simulink library "fiveDoFDynamicsCoupledFossenTurbDynamics"  (R2022a)
settings: Solver=VariableStepAuto  StartTime=0.0  StopTime=10.0  RelTol=1e-3
undefined symbols (not defined in the file): eulAng2RotMat_ul, eulDot, EulerAngle2RotMat, vcl
libraries: vrlib x7, sharedutil x3, posAng2RotMat_ul x1, elevAzimAngles x1
settings Model: Creator=jldanie5  LastModifiedBy=adabney
settings SolverCC: AlgebraicLoopSolver=TrustRegion
settings DebuggingCC: UnconnectedInputMsg=warning  UnconnectedOutputMsg=warning  UnconnectedLineMsg=warning  SFMachineParentedDataDiag=warning  ArithmeticOperatorsInVariantConditions=warning
settings SFSimCC: CustomCodeUndefinedFunction=UseInterfaceOnly

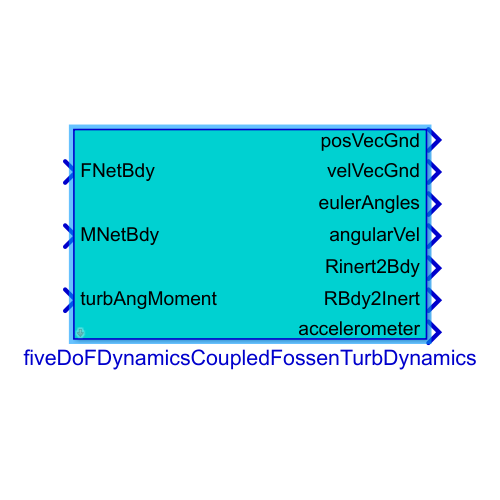
[thumbnail: Simulink's stored preview of the top-level diagram]
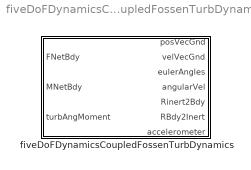
== system fiveDoFDynamicsCoupledFossenTurbDynamics ==
  fiveDoFDynamicsCoupledFossenTurbDynamics : Subsystem  VariantControl=VSS_sixDoFDynamics_sixDoFDynamicsCoupledFossenTurbDynamics  mask{MMat=vcl.M6x6_B.Value, MaMat=vcl.Ma6x6_LE.Value, rCM_B=vcl.rCM_B.Value, rB_LE=vcl.rB_LE.Value, initPos=vcl.initPosVecGnd.Value, initVel=vcl.initVelVecBdy.Value, initEulAngs=vcl.initEulAng.Value, initAngVel=vcl.initAngVelVec.Value}
      mask prompts: MMat "6x6 Mass Matrix"; MaMat "6x6 Added Mass Matrix"; rCM_B "Center of mass position vec in body frame"; rB_LE "Body frame origin position vec relative to Leading Edge"; initPos "Initial position"; initVel "Initial velocity"; initEulAngs "Initial Euler Angles"; initAngVel "Initial Angular Velocity Vec"
      mask init:
      | %Calculate Added Mass Matrices
      | S = @(v) [0 -v(3) v(2);v(3) 0 -v(1);-v(2) v(1) 0];
      | MaAdj = [eye(3) zeros(3);-S(rB_LE) eye(3)]*MaMat;
      | MTot = MMat + MaAdj;
      | MTotInv = inv(MTot);
      | 
      | %Calculate system mass and inertia
      | m = MMat(1,1);
      | J = MMat(4:6,4:6);%About Body Frame 
      | 
      | %Calculate system initial position angles
      | x = initPos(1);
      | y = initPos(2);
      | z = initPos(3);
      | R = sqrt(sum(initPos.^2));
      | el = atan2(z,sqrt(x^2+y^2));
      | az = atan2(y,x);
      | 
      | %Calculate initial spherical velocities
      | r = initEulAngs(1); sr = sin(r); cr = cos(r);
      | p = initEulAngs(2); sp = sin(p); cp = cos(p);
      | y = initEulAngs(3); sy = sin(y); cy = cos(y);
      | se = sin(el); ce = cos(el);
      | sa = sin(az); ca = cos(az);
      | 
      | %Calculate Rotation Matrices
      | Rx = [1 0 0; 0 cr sr; 0 -sr cr];
      | Ry = [cp 0 -sp; 0 1 0; sp 0 cp];
      | Rz = [cy sy 0; -sy cy 0; 0 0 1];
      | Ra = [ca sa 0; -sa ca 0; 0 0 1];
      | Re = [ce 0 -se; 0 1 0; se 0 ce];
      | Reul = Rx*Ry*Rz;
      | Rsph = Re*Ra;
      | 
      | %Calculate Initial Velocities
      | velSp = Rsph*Reul'*initVel;
      | initVelSph = velSp(2:3);
      mask DialogControl Container6 Prompt: Mass Matrices
      mask DialogControl Container4 Prompt: Point Locations
      mask DialogControl Container3 Prompt: Initial Conditions

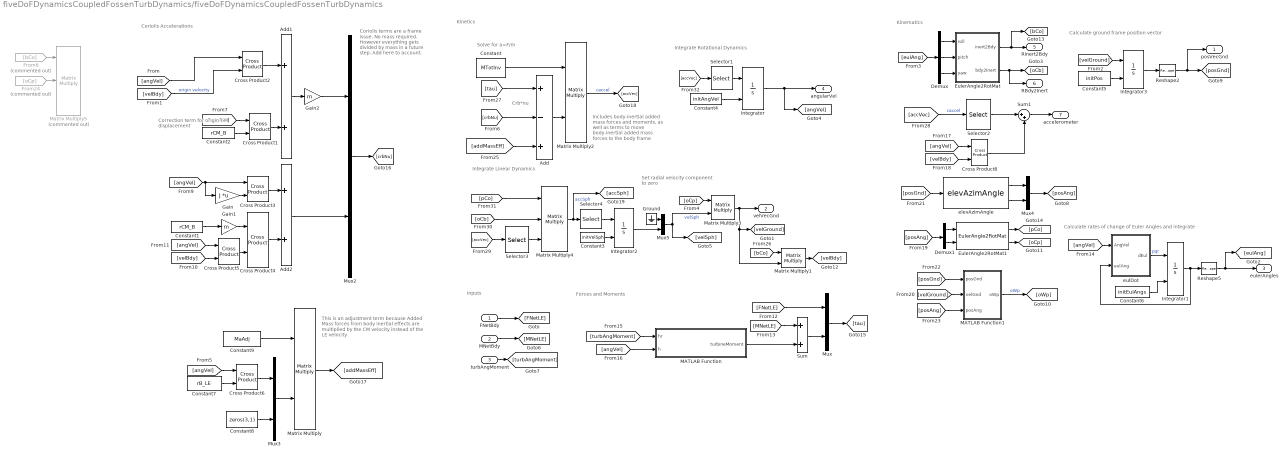
== system fiveDoFDynamicsCoupledFossenTurbDynamics/fiveDoFDynamicsCoupledFossenTurbDynamics ==
  note: Kinematics
  note: Kinetics
  note: Set radial velocity
      | component to zero
  note: Integrate Linear Dynamics
  note: Coriolis terms are a frame issue. No mass required. However everything gets divided by mass in a future step. Add here to account.
  note: Coriolis Accelerations
  note: Correction term for origin-CM displacement
  note: Forces and Moments
  note: Inputs
  note: Calculate rates of change of Euler Angles and integrate
  note: Calculate ground frame position vector
  note: Includes body-inertial added mass forces and moments,
      | as well as terms to move body-inertial added mass
      | forces to the body frame
  note: Crb*nu
  note: This is an adjustment term because Added
      | Mass forces from body inertial effects are
      | multiplied by the CM velocity instead
      | of the LE velocity
  note: Integrate Rotational Dynamics
  note: Solve for a=F/m
  FNetBdy : Inport
  MNetBdy : Inport  Port=2
  turbAngMoment : Inport  Port=3
  Add : Sum  Inputs=+-+
  Add1 : Sum
  Add2 : Sum
  Constant : Constant  Value=MTotInv  VectorParams1D=off
  Constant1 : Constant  Value=rCM_B
  Constant2 : Constant  Value=rCM_B
  Constant3 : Constant  Value=initVelSph
  Constant4 : Constant  Value=initAngVel
  Constant5 : Constant  Value=initPos
  Constant6 : Constant  Value=initEulAngs
  Constant7 : Constant  Value=rB_LE
  Constant8 : Constant  Value=zeros(3,1)
  Constant9 : Constant  Value=MaAdj
  Cross Product{1..6,8} (7 alike) : vrlib/Utilities/Cross Product
  Demux : Demux  Outputs=3
  Demux1 : Demux  Outputs=2
  EulerAngle2RotMat : Subsystem  AncestorBlock=eulAng2RotMat_ul/EulerAngle2RotMat
  EulerAngle2RotMat1 : posAng2RotMat_ul/EulerAngle2RotMat  SystemSampleTime=-1  VariantActivationTime=update diagram  Latency=0  AutoFrameSizeCalculation=off
  From24 : From  Commented=on  GotoTag=oCp
  From8 : From  Commented=on  GotoTag=bCo
  Gain : Gain  Gain=J  Multiplication=Matrix(K*u)
  Gain1 : Gain  Gain=m
  Gain2 : Gain  Gain=m
  Ground : Ground
  Integrator : Integrator  InitialConditionSource=external
  Integrator1 : Integrator  InitialConditionSource=external  InitialCondition=initEulAngs
  Integrator2 : Integrator  InitialConditionSource=external  ContinuousStateAttributes={'vA','vE'}
  Integrator3 : Integrator  InitialConditionSource=external  InitialCondition=initPos
  MATLAB Function : MATLAB Function  TreatAsAtomicUnit=on
  MATLAB Function1 : MATLAB Function  TreatAsAtomicUnit=on
  Matrix Multiply{,1..3} (4 alike) : Product  Multiplication=Matrix(*)
  Matrix Multiply4 : Product  Inputs=3  Multiplication=Matrix(*)
  Matrix Multiply5 : Product  Commented=on  Inputs=3  Multiplication=Matrix(*)
  Mux{,2..5} (5 alike) : Mux  Inputs=2
  Reshape2 : Reshape  OutputDimensionality=Column vector (2-D)
  Reshape5 : Reshape  OutputDimensionality=Column vector (2-D)
  Selector1 : Selector  InputPortWidth=6  IndexOptions=Index vector (dialog)  Indices=[4 5 6]  OutputSizes=1
  Selector2 : Selector  InputPortWidth=6  IndexOptions=Index vector (dialog)  Indices=[1 2 3]  OutputSizes=1
  Selector3 : Selector  InputPortWidth=6  IndexOptions=Index vector (dialog)  Indices=[1 2 3]  OutputSizes=1
  Selector4 : Selector  InputPortWidth=3  IndexOptions=Index vector (dialog)  Indices=[2 3]  OutputSizes=1
  Sum : Sum
  Sum1 : Sum  Inputs=|++
  elevAzimAngle : elevAzimAngles/elevAzimAngle  SystemSampleTime=-1  VariantActivationTime=update diagram  Latency=0  AutoFrameSizeCalculation=off
  eulDot : Subsystem  AncestorBlock=eulDot/eulDot
  posVecGnd : Outport  VectorParamsAs1DForOutWhenUnconnected=off
  velVecGnd : Outport  Port=2  VectorParamsAs1DForOutWhenUnconnected=off
  eulerAngles : Outport  Port=3  VectorParamsAs1DForOutWhenUnconnected=off
  angularVel : Outport  Port=4  VectorParamsAs1DForOutWhenUnconnected=off
  Rinert2Bdy : Outport  Port=5  VectorParamsAs1DForOutWhenUnconnected=off
  RBdy2Inert : Outport  Port=6  VectorParamsAs1DForOutWhenUnconnected=off
  accelerometer : Outport  Port=7  VectorParamsAs1DForOutWhenUnconnected=off
  wires:
  MATLAB Function/1(turbineMoment) -> Sum/2
  [turbAngMoment] -> MATLAB Function/1(hr)
  [angVel] -> MATLAB Function/2(h)
  Sum/1 -> Mux/2
  turbAngMoment/1 -> [turbAngMoment]
  [MNetLE] -> Sum/1
  [FNetLE] -> Mux/1
  MNetBdy/1 -> [MNetLE]
  FNetBdy/1 -> [FNetLE]
  Add/1 -> Matrix Multiply2/2
  Add2/1 -> Mux2/2
  Cross Product4/1 -> Add2/2
  Cross Product5/1 -> Cross Product4/2
  [angVel] -> Cross Product5/1
  [velBdy] -> Cross Product5/2
  Gain1/1 -> Cross Product4/1
  Constant1/1 -> Gain1/1
  Gain/1 -> Cross Product3/2
  [angVel] -> Gain/1, Cross Product3/1
  Mux2/1 -> [crbNu]
  EulerAngle2RotMat/1(inert2Bdy) -> [bCo], Rinert2Bdy/1
  [velGround] -> Integrator3/1
  Integrator/1 -> angularVel/1, [angVel]
  Reshape5/1 -> [eulAng], eulerAngles/1
  Constant6/1 -> Integrator1/2
  Integrator1/1 -> eulDot/2(eulAng), Reshape5/1
  eulDot/1(dEul) -> Integrator1/1  "pqr"
  [eulAng] -> Demux/1
  Constant5/1 -> Integrator3/2
  Demux/2 -> EulerAngle2RotMat/2(pitch)
  Reshape2/1 -> posVecGnd/1, [posGnd]
  EulerAngle2RotMat/2(bdy2Inert) -> [oCb], RBdy2Inert/1
  Demux/1 -> EulerAngle2RotMat/1(roll)
  Demux/3 -> EulerAngle2RotMat/3(yaw)
  Integrator3/1 -> Reshape2/1
  Constant4/1 -> Integrator/2
  Matrix Multiply2/1 -> [accVec]  "caccel"
  Constant/1 -> Matrix Multiply2/1
  Mux/1 -> [tau]
  Demux1/2 -> EulerAngle2RotMat1/2
  Demux1/1 -> EulerAngle2RotMat1/1
  [posAng] -> Demux1/1
  EulerAngle2RotMat1/1 -> [pCo]
  [velGround] -> MATLAB Function1/2(velGnd)
  [posGnd] -> elevAzimAngle/1
  elevAzimAngle/1 -> Mux4/1
  elevAzimAngle/2 -> Mux4/2
  Mux4/1 -> [posAng]
  [posGnd] -> MATLAB Function1/1(posGnd)
  [posAng] -> MATLAB Function1/3(posAng)
  MATLAB Function1/1(oWp) -> [oWp]  "oWp"
  EulerAngle2RotMat1/2 -> [oCp]
  Cross Product3/1 -> Add2/1
  [tau] -> Add/1
  Constant2/1 -> Cross Product1/2
  Cross Product1/1 -> Add1/2
  Add1/1 -> Gain2/1
  [angVel] -> Cross Product1/1
  [velBdy] -> Cross Product2/2  "origin velocity"
  Gain2/1 -> Mux2/1
  Cross Product2/1 -> Add1/1
  [angVel] -> Cross Product6/1
  Constant8/1 -> Mux3/2
  Constant9/1 -> Matrix Multiply/1
  Mux3/1 -> Matrix Multiply/2
  Constant7/1 -> Cross Product6/2
  Matrix Multiply/1 -> [addMassEff]
  Cross Product6/1 -> Mux3/1
  [addMassEff] -> Add/3
  [crbNu] -> Add/2
  Selector2/1 -> Sum1/1
  Sum1/1 -> accelerometer/1
  [accVec] -> Selector2/1  "caccel"
  Cross Product8/1 -> Sum1/2
  [angVel] -> Cross Product8/1
  [velBdy] -> Cross Product8/2
  [accVec] -> Selector3/1
  Selector3/1 -> Matrix Multiply4/3
  [oCb] -> Matrix Multiply4/2
  [pCo] -> Matrix Multiply4/1
  Matrix Multiply4/1 -> [accSph], Selector4/1  "accSph"
  Selector4/1 -> Integrator2/1
  Constant3/1 -> Integrator2/2
  Integrator2/1 -> Mux5/2
  Matrix Multiply3/1 -> velVecGnd/1, Matrix Multiply1/2, [velGround]
  Ground/1 -> Mux5/1
  [oCp] -> Matrix Multiply3/1
  Matrix Multiply1/1 -> [velBdy]
  [bCo] -> Matrix Multiply1/1
  Mux5/1 -> [velSph], Matrix Multiply3/2  "velSph"
  Selector1/1 -> Integrator/1
  [accVec] -> Selector1/1
  [angVel] -> Cross Product2/1
  [angVel] -> eulDot/1(AngVel)
  From8/1 -> Matrix Multiply5/1
  From24/1 -> Matrix Multiply5/2

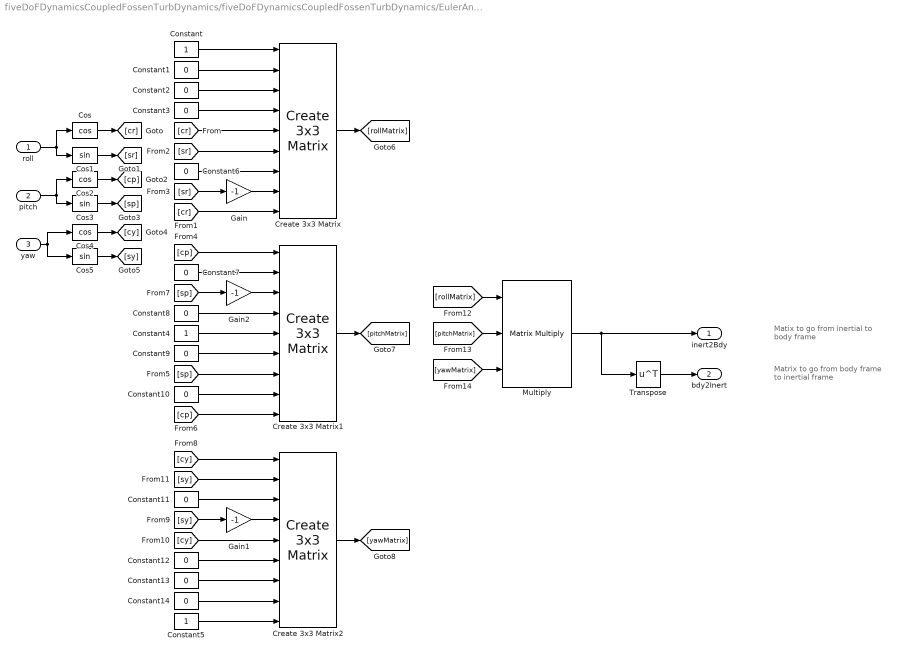
== system fiveDoFDynamicsCoupledFossenTurbDynamics/fiveDoFDynamicsCoupledFossenTurbDynamics/EulerAngle2RotMat ==
  note: Matrix to go from body
      | frame to inertial frame
  note: Matix to go from
      | inertial to body frame
  roll : Inport
  pitch : Inport  Port=2
  yaw : Inport  Port=3
  Constant : Constant
  Constant{1..3,6..14} (12 alike) : Constant  Value=0
  Constant4 : Constant
  Constant5 : Constant
  Cos : Trigonometry  Operator=cos
  Cos1 : Trigonometry
  Cos2 : Trigonometry  Operator=cos
  Cos3 : Trigonometry
  Cos4 : Trigonometry  Operator=cos
  Cos5 : Trigonometry
  Create 3x3 Matrix : sharedutil/Create 3x3 Matrix  aMode=aMode
      settings: SourceProductBaseCode=AE,PW,DR,MT,VE
  Create 3x3 Matrix1 : sharedutil/Create 3x3 Matrix  aMode=aMode
      settings: SourceProductBaseCode=AE,PW,DR,MT,VE
  Create 3x3 Matrix2 : sharedutil/Create 3x3 Matrix  aMode=aMode
      settings: SourceProductBaseCode=AE,PW,DR,MT,VE
  Gain : Gain  Gain=-1
  Gain1 : Gain  Gain=-1
  Gain2 : Gain  Gain=-1
  Multiply : Product  Inputs=3  Multiplication=Matrix(*)
  Transpose : Math  Operator=transpose  SignedPower=on
  inert2Bdy : Outport  VectorParamsAs1DForOutWhenUnconnected=off
  bdy2Inert : Outport  Port=2  VectorParamsAs1DForOutWhenUnconnected=off
  wires:
  roll/1 -> Cos/1, Cos1/1
  Cos/1 -> [cr]
  Cos1/1 -> [sr]
  pitch/1 -> Cos3/1, Cos2/1
  yaw/1 -> Cos4/1, Cos5/1
  Cos2/1 -> [cp]
  Cos3/1 -> [sp]
  Cos4/1 -> [cy]
  Cos5/1 -> [sy]
  Constant/1 -> Create 3x3 Matrix/1
  Constant1/1 -> Create 3x3 Matrix/2
  [cr] -> Create 3x3 Matrix/5
  [cr] -> Create 3x3 Matrix/9
  [sr] -> Gain/1
  Constant3/1 -> Create 3x3 Matrix/4
  Constant2/1 -> Create 3x3 Matrix/3
  Constant6/1 -> Create 3x3 Matrix/7
  [sr] -> Create 3x3 Matrix/6
  Create 3x3 Matrix/1 -> [rollMatrix]
  Constant4/1 -> Create 3x3 Matrix1/5
  Constant5/1 -> Create 3x3 Matrix2/9
  Constant7/1 -> Create 3x3 Matrix1/2
  Constant8/1 -> Create 3x3 Matrix1/4
  Constant9/1 -> Create 3x3 Matrix1/6
  Constant10/1 -> Create 3x3 Matrix1/8
  Constant11/1 -> Create 3x3 Matrix2/3
  Constant12/1 -> Create 3x3 Matrix2/6
  Constant13/1 -> Create 3x3 Matrix2/7
  Constant14/1 -> Create 3x3 Matrix2/8
  [cp] -> Create 3x3 Matrix1/1
  [cp] -> Create 3x3 Matrix1/9
  [sp] -> Gain2/1
  [sp] -> Create 3x3 Matrix1/7
  [cy] -> Create 3x3 Matrix2/1
  [cy] -> Create 3x3 Matrix2/5
  [sy] -> Gain1/1
  Create 3x3 Matrix1/1 -> [pitchMatrix]
  Create 3x3 Matrix2/1 -> [yawMatrix]
  Multiply/1 -> Transpose/1, inert2Bdy/1
  Transpose/1 -> bdy2Inert/1
  [rollMatrix] -> Multiply/1
  [yawMatrix] -> Multiply/3
  [pitchMatrix] -> Multiply/2
  Gain/1 -> Create 3x3 Matrix/8
  Gain1/1 -> Create 3x3 Matrix2/4
  [sy] -> Create 3x3 Matrix2/2
  Gain2/1 -> Create 3x3 Matrix1/3

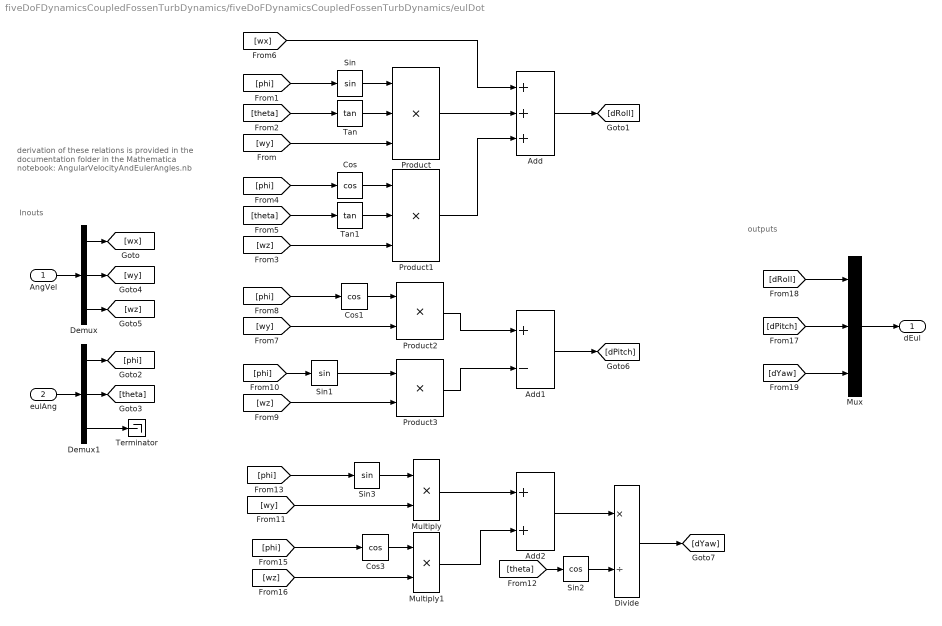
== system fiveDoFDynamicsCoupledFossenTurbDynamics/fiveDoFDynamicsCoupledFossenTurbDynamics/eulDot ==
  note: derivation of these relations is provided in
      | the documentation folder in the Mathematica
      | notebook: AngularVelocityAndEulerAngles.nb
  note: outputs
  note: Inouts
  AngVel : Inport
  eulAng : Inport  Port=2
  Add : Sum  Inputs=+++
  Add1 : Sum  Inputs=+-
  Add2 : Sum
  Cos : Trigonometry  Operator=cos
  Cos1 : Trigonometry  Operator=cos
  Cos3 : Trigonometry  Operator=cos
  Demux : Demux  Outputs=3
  Demux1 : Demux  Outputs=3
  Divide : Product  Inputs=*/
  Multiply : Product
  Multiply1 : Product
  Mux : Mux  Inputs=3
  Product : Product  Inputs=3
  Product1 : Product  Inputs=3
  Product2 : Product
  Product3 : Product
  Sin : Trigonometry
  Sin1 : Trigonometry
  Sin2 : Trigonometry  Operator=cos
  Sin3 : Trigonometry
  Tan : Trigonometry  Operator=tan
  Tan1 : Trigonometry  Operator=tan
  Terminator : Terminator
  dEul : Outport  VectorParamsAs1DForOutWhenUnconnected=off
  wires:
  Demux1/3 -> Terminator/1
  Sin/1 -> Product/1
  Tan/1 -> Product/2
  [wy] -> Product/3
  [phi] -> Sin/1
  [theta] -> Tan/1
  Cos/1 -> Product1/1
  Tan1/1 -> Product1/2
  [wz] -> Product1/3
  [theta] -> Tan1/1
  [phi] -> Cos/1
  Product/1 -> Add/2
  [wx] -> Add/1
  Product1/1 -> Add/3
  Add/1 -> [dRoll]
  [phi] -> Cos1/1
  Cos1/1 -> Product2/1
  [wy] -> Product2/2
  Sin1/1 -> Product3/1
  [wz] -> Product3/2
  [phi] -> Sin1/1
  Product2/1 -> Add1/1
  Product3/1 -> Add1/2
  [theta] -> Sin2/1
  [phi] -> Sin3/1
  Sin2/1 -> Divide/2
  Sin3/1 -> Multiply/1
  [wy] -> Multiply/2
  [phi] -> Cos3/1
  Cos3/1 -> Multiply1/1
  [wz] -> Multiply1/2
  Multiply/1 -> Add2/1
  Multiply1/1 -> Add2/2
  Demux/1 -> [wx]
  Demux/2 -> [wy]
  Demux/3 -> [wz]
  AngVel/1 -> Demux/1
  eulAng/1 -> Demux1/1
  Demux1/1 -> [phi]
  Demux1/2 -> [theta]
  Add1/1 -> [dPitch]
  Add2/1 -> Divide/1
  [dPitch] -> Mux/2
  [dRoll] -> Mux/1
  [dYaw] -> Mux/3
  Mux/1 -> dEul/1
  Divide/1 -> [dYaw]

== matlab function fiveDoFDynamicsCoupledFossenTurbDynamics/MATLAB Function ==
  data: hr input; turbineMoment output; h input
function turbineMoment = fcn(hr,h)
    turbineMoment = [hr(2)*h(3)-hr(3)*h(2) ;...
                     hr(3)*h(1)-hr(1)*h(3) ;...
                     hr(1)*h(2)-hr(2)*h(1) ];
    
end

== matlab function fiveDoFDynamicsCoupledFossenTurbDynamics/MATLAB Function1 ==
  data: posGnd input; oWp output; velGnd input; posAng input
function oWp = fcn(posGnd,velGnd,posAng)
%Load Values
x = posGnd(1);
y = posGnd(2);
z = posGnd(3);
xDot = velGnd(1);
yDot = velGnd(2);
zDot = velGnd(3);
theta = posAng(1);
phi = posAng(2);

%Calculate Position Angle Derivatives
dTheta = cos(theta)^2*...
    (zDot/sqrt(x^2+y^2)-z/(x^2+y^2)^(3/2)*(x*xDot+y*yDot));
dPhi = cos(phi)^2*(yDot/x-xDot*y/x^2);

%Calculate Angular Veloicty of the spherical frame
oWp = [-sin(theta)*dPhi;dTheta;cos(theta)*dPhi];
